simulink model "task1_lab9"  (R2021a)
settings: Solver=VariableStepAuto  StartTime=0.0  StopTime=10.0  RelTol=1e-3
settings Model: Creator=reemb  LastModifiedBy=reemb

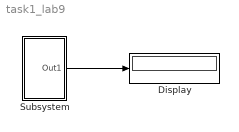
== system task1_lab9 ==
  Display : Display
  Subsystem : Subsystem  TreatAsAtomicUnit=on
  wires:
  Subsystem/1(Out1) -> Display/1

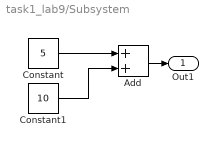
== system task1_lab9/Subsystem ==
  Add : Sum
  Constant : Constant  Value=5
  Constant1 : Constant  Value=10
  Out1 : Outport
  wires:
  Constant1/1 -> Add/2
  Constant/1 -> Add/1
  Add/1 -> Out1/1
